simulink model "ChildApp"  (R2023b)
settings: Solver=FixedStepAuto  StartTime=0.0  StopTime=inf  RelTol=1e-3
undefined symbols (not defined in the file): a, b, child, Fuzzy_Logic_out, Sound_level, x_accl, y, y_accl, z, z_accl
libraries: androiduilib x9, androidcommunicationlib x4, androidsensorlib x3, androidaudiovideolib x3, fuzblock x1
settings Model: Creator=91940  LastModifiedBy=Dell
settings OptimizationCC: EnhancedBackFolding=on  PassReuseOutputArgsAs=Individual arguments  ZeroExternalMemoryAtStartup=off  ZeroInternalMemoryAtStartup=off  MaxStackSize=64  OptimizeBlockOrder=speed  DifferentSizesBufferReuse=on  OptimizationCustomize=off  EfficientTunableParamExpr=on
settings DebuggingCC: ParameterTunabilityLossMsg=error
settings HardwareCC: ProdBitPerPointer=32  ProdBitPerSizeT=32  ProdBitPerPtrDiffT=32  ProdLargestAtomicInteger=Long  ProdLargestAtomicFloat=Double  ProdWordSize=32  ProdHWDeviceType=ARM Compatible->ARM Cortex  UseEmbeddedCoderFeatures=off  UseSimulinkCoderFeatures=off
settings ModelReferenceCC: EnableRefExpFcnMdlSchedulingChecks=on
settings SFSimCC: MATLABDynamicMemAlloc=off
settings RTWCC: Description=Embedded Coder  SystemTargetFile=ert.tlc  HardwareBoard=Android Device  TLCOptions="-aInlineSetEventsForThisBaseRateFcn=TLC_FALSE -aSuppressMultiTaskScheduler=TLC_FALSE  -aRateBasedStepFcn=0"  TemplateMakefile=ert_default_tmf  RTWVerbose=off  Toolchain=Android SDK/NDK Tools
settings CodeAppCC: ForceParamTrailComments=on  IgnoreCustomStorageClasses=off  OperatorAnnotations=on  SimulinkDataObjDesc=on  SFDataObjDesc=on  InsertBlockDesc=on
settings ERTTargetCC: SupportNonInlinedSFcns=on

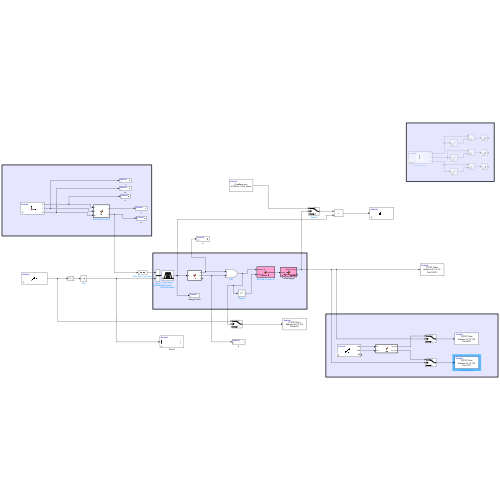
[thumbnail: Simulink's stored preview of the top-level diagram]
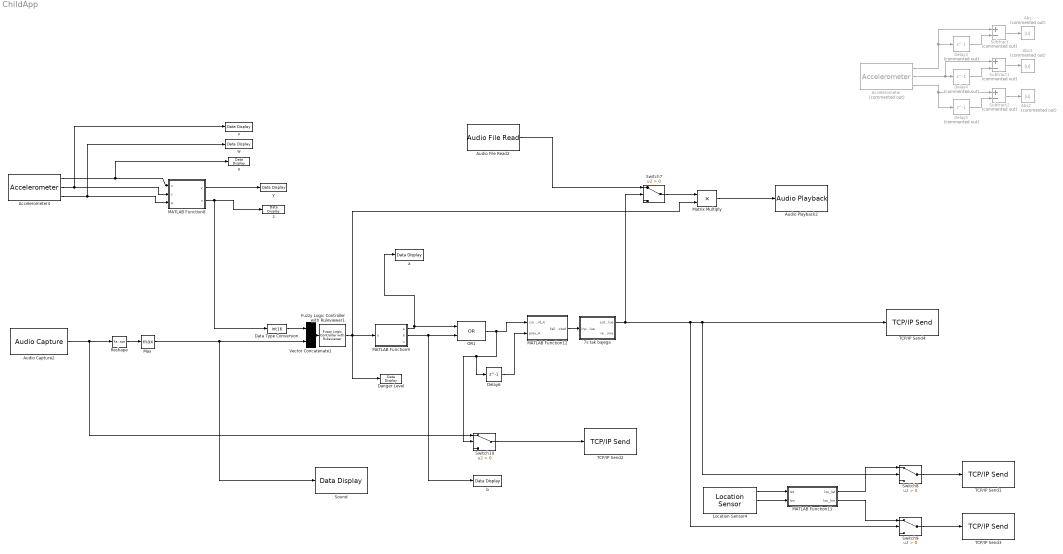
== system ChildApp ==
  7s tak bajega : MATLAB Function  TreatAsAtomicUnit=on
  Abs : Abs  Commented=on  SaturateOnIntegerOverflow=off
  Abs1 : Abs  Commented=on  SaturateOnIntegerOverflow=off
  Abs2 : Abs  Commented=on  SaturateOnIntegerOverflow=off
  Accelerometer : androidsensorlib/Accelerometer  Commented=on  OutputVector=off  SampleTime=0.1  BlockPlatform=Android
  Accelerometer4 : androidsensorlib/Accelerometer  OutputVector=off  SampleTime=0.1  BlockPlatform=Android
  Audio Capture2 : androidaudiovideolib/Audio Capture  SampleFreq=44100  FrameSize=4410  SampleTime=0.1  SimulateUsing=Code generation  DeviceStr=0  QueueDuration=0  BlockPlatform=Android  AudioSamplingFreq=44100
  Audio File Read2 : androidaudiovideolib/Audio File Read  FileName=C:\Users\Dell\Downloads\FinalBeep.wav  FrameSize=4410
  Audio Playback2 : androidaudiovideolib/Audio Playback  SampleFreq=44100  AudioSamplingFreq=44100  SampleTime=0.1  DeviceStr=0  QueueDuration=0  BlockPlatform=Android
  Danger Level : androiduilib/Data Display  DataDisplayId=child/Fuzzy_Logic_out  Format=Float  Precision=6  SimulateUsing=Code generation  blockPlatform=Android
  Data Type Conversion : DataTypeConversion  OutDataTypeStr=int16  SaturateOnIntegerOverflow=off  RndMeth=Floor
  Delay3 : Delay  Commented=on  DelayLength=1  InitialCondition=0
  Delay4 : Delay  Commented=on  DelayLength=1  InitialCondition=0
  Delay5 : Delay  Commented=on  DelayLength=1  InitialCondition=0
  Delay6 : Delay  DelayLength=1  InitialCondition=0
  Fuzzy Logic Controller with Ruleviewer1 : fuzblock/Fuzzy Logic  Controller  with Ruleviewer  fismatrix=fuzzyyy  Ts=0.1
  Location Sensor4 : androidsensorlib/Location Sensor  OutputVector=off  SampleTime=0.1  BlockPlatform=Android
  MATLAB Function11 : MATLAB Function  TreatAsAtomicUnit=on
  MATLAB Function12 : MATLAB Function  TreatAsAtomicUnit=on
  MATLAB Function8 : MATLAB Function  TreatAsAtomicUnit=on
  MATLAB Function9 : MATLAB Function  TreatAsAtomicUnit=on
  Matrix Multiply : Product  OutDataTypeStr=int16
  Max : MinMax  Function=max
  OR1 : Logic  Operator=OR  IconShape=distinctive  AllPortsSameDT=off  OutDataTypeStr=boolean
  Reshape : Reshape
  Sound : androiduilib/Data Display  DataDisplayId=child/Sound_level  Format=Float  Precision=6  SimulateUsing=Code generation  blockPlatform=Android
  Subtract : Sum  Commented=on  Inputs=+-
  Subtract1 : Sum  Commented=on  Inputs=+-
  Subtract2 : Sum  Commented=on  Inputs=+-
  Switch{7..10} (4 alike) : Switch  Criteria=u2 > Threshold  SaturateOnIntegerOverflow=off  InputSameDT=off
  TCP/IP Send1 : androidcommunicationlib/TCP//IP Send  TCPSendId=child/TCP//IP_Send1  Mode_=Client  LocalServerPort_=25000  RemoteAddr_=10.7.9.132  RemoteServerPort_=8070  ClientPortBindingSelection_=off  ClientPortToBind_=35000  BlockingMode_=off  BlockTimeout_=0.1
  TCP/IP Send2 : androidcommunicationlib/TCP//IP Send  TCPSendId=child/TCP//IP_Send2  Mode_=Client  LocalServerPort_=25000  RemoteAddr_=10.7.9.132  RemoteServerPort_=9070  ClientPortBindingSelection_=off  ClientPortToBind_=35000  BlockingMode_=off  BlockTimeout_=0.1
  TCP/IP Send3 : androidcommunicationlib/TCP//IP Send  TCPSendId=child/TCP//IP_Send3  Mode_=Client  LocalServerPort_=25000  RemoteAddr_=10.7.9.132  RemoteServerPort_=7070  ClientPortBindingSelection_=off  ClientPortToBind_=35000  BlockingMode_=off  BlockTimeout_=0.1
  TCP/IP Send4 : androidcommunicationlib/TCP//IP Send  TCPSendId=child/TCP//IP_Send4  Mode_=Client  LocalServerPort_=25000  RemoteAddr_=10.7.9.132  RemoteServerPort_=10070  ClientPortBindingSelection_=off  ClientPortToBind_=35000  BlockingMode_=off  BlockTimeout_=0.1
  Vector Concatenate1 : Concatenate
  a : androiduilib/Data Display  DataDisplayId=child/a  Format=Float  Precision=6  SimulateUsing=Code generation  blockPlatform=Android
  b : androiduilib/Data Display  DataDisplayId=child/b  Format=Float  Precision=6  SimulateUsing=Code generation  blockPlatform=Android
  u : androiduilib/Data Display  DataDisplayId=child/x_accl  Format=Float  Precision=6  SimulateUsing=Code generation  blockPlatform=Android
  v : androiduilib/Data Display  DataDisplayId=child/y_accl  Format=Float  Precision=6  SimulateUsing=Code generation  blockPlatform=Android
  w : androiduilib/Data Display  DataDisplayId=child/z_accl  Format=Float  Precision=6  SimulateUsing=Code generation  blockPlatform=Android
  y : androiduilib/Data Display  DataDisplayId=child/y  Format=Float  Precision=6  SimulateUsing=Code generation  blockPlatform=Android
  z : androiduilib/Data Display  DataDisplayId=child/z  Format=Float  Precision=6  SimulateUsing=Code generation  blockPlatform=Android
  wires:
  MATLAB Function8/1(y) -> y/1
  MATLAB Function8/2(z) -> z/1, Data Type Conversion/1
  Fuzzy Logic Controller with Ruleviewer1/1 -> Matrix Multiply/2, MATLAB Function9/1(u), Danger Level/1
  MATLAB Function9/1(a) -> OR1/1, a/1
  MATLAB Function9/2(b) -> b/1, OR1/2
  MATLAB Function11/2(loc_lon) -> Switch9/1
  Location Sensor4/2 -> MATLAB Function11/2(lon)
  MATLAB Function11/1(loc_lat) -> Switch8/1
  Switch8/1 -> TCP/IP Send1/1
  Location Sensor4/1 -> MATLAB Function11/1(lat)
  Switch10/1 -> TCP/IP Send2/1
  Audio Capture2/1 -> Switch10/1, Reshape/1
  Reshape/1 -> Max/1
  Max/1 -> Sound/1, Vector Concatenate1/2
  Vector Concatenate1/1 -> Fuzzy Logic Controller with Ruleviewer1/1
  Data Type Conversion/1 -> Vector Concatenate1/1
  Audio File Read2/1 -> Switch7/1
  Delay5/1 -> Subtract2/2
  Subtract1/1 -> Abs1/1
  Subtract/1 -> Abs/1
  Delay3/1 -> Subtract/2
  Subtract2/1 -> Abs2/1
  Accelerometer/1 -> Subtract/1, Delay3/1
  Accelerometer/2 -> Subtract1/1, Delay4/1
  Accelerometer/3 -> Subtract2/1, Delay5/1
  Delay4/1 -> Subtract1/2
  Accelerometer4/1 -> u/1, MATLAB Function8/1(u)
  Accelerometer4/2 -> MATLAB Function8/2(v), v/1
  Accelerometer4/3 -> MATLAB Function8/3(w), w/1
  Matrix Multiply/1 -> Audio Playback2/1
  Switch7/1 -> Matrix Multiply/1
  OR1/1 -> Switch10/2, Delay6/1, MATLAB Function12/1(current_A)
  MATLAB Function12/1(fall_detected) -> 7s tak bajega/1(input_value)
  Delay6/1 -> MATLAB Function12/2(prev_A)
  7s tak bajega/1(output_value) -> Switch8/2, TCP/IP Send4/1, Switch9/2, Switch7/2
  Switch9/1 -> TCP/IP Send3/1

== matlab function ChildApp/MATLAB Function8 ==
  data: y output; u input; v input; w input; z output
function [y,z] = fcn(u,v,w)

z=(u^2+v^2+w^2)^(1/2);

if (z>28)
    y=1;
    z=z/15;
else
  y=0;
  z=z/15;
end

== matlab function ChildApp/MATLAB Function9 ==
  data: u input; a output; b output; c output
function [a,b,c] = fcn(u)

if u>6
    a=1;
    b=0;
    c=0;
else 
    if u>4
        a=0;
        c=0;
        b=1;
    else
        a=0;
        b=0;
        c=1;
    end
end

== matlab function ChildApp/MATLAB Function11 ==
  data: lat input; loc_lat output; lon input; loc_lon output
function [loc_lat,loc_lon]= fcn(lat, lon)
 % Haversine formula to calculate distance between two points on Earth
 %   R = 6371; % Earth's radius in kilometers
  %   radius = 0.1;
    % lat1_rad = deg2rad(23.210406);
 %    lon1_rad = deg2rad(72.683669);
   %  lat2_rad = deg2rad(lat);
     %lon2_rad = deg2rad(lon);
  %   dlat = lat2_rad - lat1_rad;
    % dlon = lon2_rad - lon1_rad;
  %   a = sin(dlat/2)^2 + cos(lat1_rad) * cos(lat2_rad) * sin(dlon/2)^2;
    % c = 2 * atan2(sqrt(a), sqrt(1-a));
  %   distance = R * c;
    % z = distance;
    
    loc_lat= deg2rad(lat);
    loc_lon=deg2rad(lon);

    % Check if the distance is greater than the specified radius
   % if distance > radius
   %     y = 1; % Point is outside the specified radius
   % else
    %    y = 0; % Point is inside or on the specified radius
   % end

== matlab function ChildApp/MATLAB Function12 ==
  data: current_A input; fall_detected output; prev_A input
function fall_detected = detect_fall(current_A, prev_A)
    % Check for a change in A (current A is true and prev A is false)

    if current_A && ~prev_A
        fallDetectedState = true;
    else
        fallDetectedState = false;
    end
    
    fall_detected = fallDetectedState;
end

== matlab function ChildApp/7s tak bajega ==
  data: input_value input; output_value output; remaining_time output
function [output_value, remaining_time] = true_for_7_seconds(input_value)
    % Define a persistent variable to store the timestamp when input becomes true
    persistent true_timestamp
    
    % Initialize the persistent variable if input becomes true
    if input_value
        true_timestamp = tic;  % Record the current time
    end
    
    % Check if 5 seconds have passed since the input became true
    if ~isempty(true_timestamp) && toc(true_timestamp) <= 7
        output_value = true;
        remaining_time = 7 - toc(true_timestamp);
    else
        % Reset the persistent variables and output 'false'
        output_value = false;
        remaining_time = 0;
    end
end
